simulink model "probl6"  (R2020b)
settings: Solver=VariableStepAuto  StartTime=0.0  StopTime=10.0  RelTol=1e-3
settings Model: Creator=Admin  LastModifiedBy=Admin

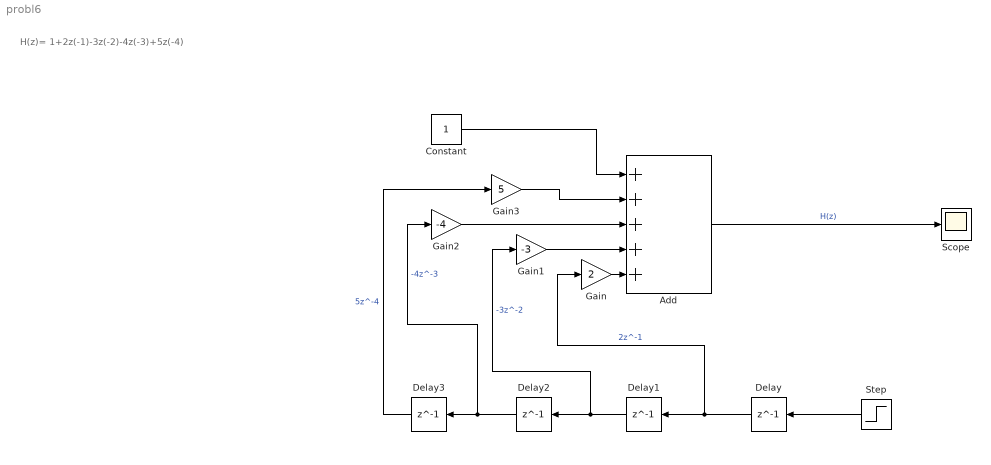
== system probl6 ==
  note: H(z)= 1+2z(-1)-3z(-2)-4z(-3)+5z(-4)
  Add : Sum  Inputs=+++++
  Constant : Constant
  Delay{,1..3} (4 alike) : Delay  DelayLength=1
  Gain : Gain  Gain=2
  Gain1 : Gain  Gain=-3
  Gain2 : Gain  Gain=-4
  Gain3 : Gain  Gain=5
  Scope : Scope
  Step : Step  SampleTime=0
  wires:
  Constant/1 -> Add/1
  Delay/1 -> Gain/1, Delay1/1  "2z^-1"
  Delay2/1 -> Gain2/1, Delay3/1  "-4z^-3"
  Delay3/1 -> Gain3/1  "5z^-4"
  Gain3/1 -> Add/2
  Add/1 -> Scope/1  "H(z)"
  Gain2/1 -> Add/3
  Delay1/1 -> Gain1/1, Delay2/1  "-3z^-2"
  Gain1/1 -> Add/4
  Step/1 -> Delay/1
  Gain/1 -> Add/5
